simulink model "DYNctl_ver4_etud_obfusc2015"  (R2015a)
settings: Solver=ode45  StartTime=0.0  StopTime=tfin  FixedStep=0.001  RelTol=1e-09
values from neighbouring files (symbols this model uses):
  A = [line1;line2;line3;line4;line5]    [sm_7.m]
  B = [m0_3x3; m0_3x3; m0_2x3; m0_2x3; mCV_3x3]    [sm_7.m]
  C = [mTTdef m0_3x3 m0_3x4 m0_3x3 ... (first row only)    [sm_7.m]
  D = zeros(7,3)    [sm_7.m]
undefined symbols (not defined in the file or in its folder): ae0, ae1, ae2, ae3, as0, as1, as2, as3, be1, C_prime, D_prime, ia_e, ib_e, ic_e, phi_e, TABC_trans, TDEF_trans, theta_e, va_e, vb_e, vc_e, vx_s_e, vy_s_e, vz_e, w_phi_e, w_theta_e, x_s_e, y_s_e, z_e, za_e, zb_e, zc_e, zd_e, ze_e, zf_e
settings Model: CovSFcnEnable=off  Creator=delafontaine  LastModifiedBy=Sytten
settings SolverCC: AlgebraicLoopSolver=LineSearch
settings DataIOCC: SignalLoggingSaveFormat=ModelDataLogs
settings DebuggingCC: UnderspecifiedInitializationDetection=Classic  MergeDetectMultiDrivingBlocksExec=none  MultiTaskDSMMsg=warning  MultiTaskCondExecSysMsg=none

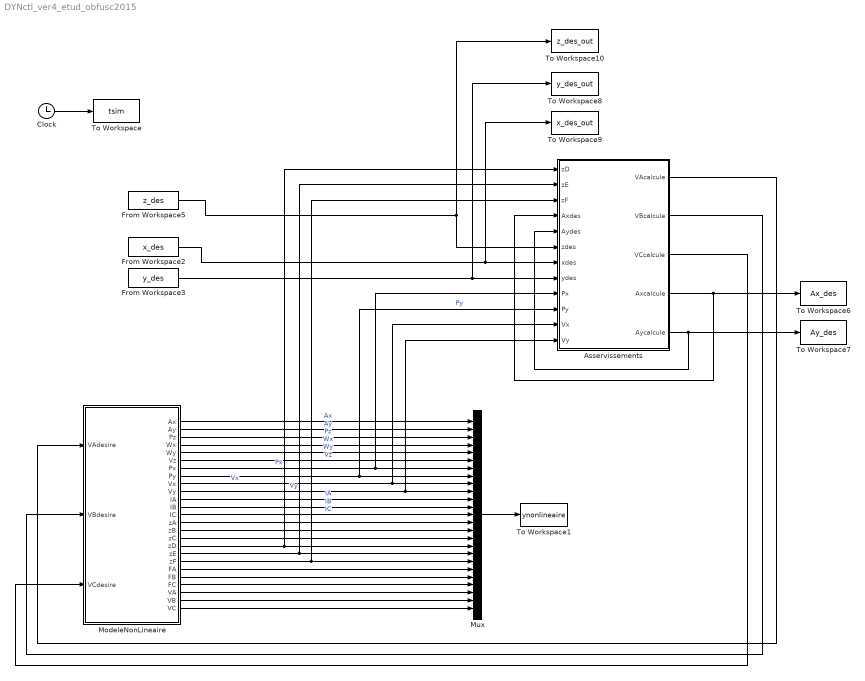
== system DYNctl_ver4_etud_obfusc2015 ==
  Asservissements : Subsystem
      mask help: Simulink:masks:GenSFuncDesc_MD
      mask Help: eval('feval(''rtwprivate'',''rtwhelpview'',''rtw_sfcn_block'')');
  Clock : Clock
  From Workspace2 : FromWorkspace  VariableName=x_des  SampleTime=0  Interpolate=off  OutputAfterFinalValue=Holding final value
  From Workspace3 : FromWorkspace  VariableName=y_des  SampleTime=0  Interpolate=off  OutputAfterFinalValue=Holding final value
  From Workspace5 : FromWorkspace  VariableName=z_des  SampleTime=0  Interpolate=off  OutputAfterFinalValue=Holding final value
  ModeleNonLineaire : Subsystem
      mask help: Simulink:masks:GenSFuncDesc_MD
      mask Help: eval('feval(''rtwprivate'',''rtwhelpview'',''rtw_sfcn_block'')');
  Mux : Mux  Inputs=25
  To Workspace : ToWorkspace  VariableName=tsim  SampleTime=-1
  To Workspace1 : ToWorkspace  VariableName=ynonlineaire  SampleTime=-1
  To Workspace10 : ToWorkspace  VariableName=z_des_out  SampleTime=-1
  To Workspace6 : ToWorkspace  VariableName=Ax_des  SampleTime=-1
  To Workspace7 : ToWorkspace  VariableName=Ay_des  SampleTime=-1
  To Workspace8 : ToWorkspace  VariableName=y_des_out  SampleTime=-1
  To Workspace9 : ToWorkspace  VariableName=x_des_out  SampleTime=-1
  wires:
  Mux/1 -> To Workspace1/1
  Clock/1 -> To Workspace/1
  From Workspace5/1 -> Asservissements/6(zdes), To Workspace10/1
  ModeleNonLineaire/1(Ax) -> Mux/1  "Ax"
  ModeleNonLineaire/2(Ay) -> Mux/2  "Ay"
  ModeleNonLineaire/3(Pz) -> Mux/3  "Pz"
  ModeleNonLineaire/4(Wx) -> Mux/4  "Wx"
  ModeleNonLineaire/5(Wy) -> Mux/5  "Wy"
  ModeleNonLineaire/6(Vz) -> Mux/6  "Vz"
  ModeleNonLineaire/7(Px) -> Asservissements/9(Px), Mux/7  "Px"
  ModeleNonLineaire/8(Py) -> Asservissements/10(Py), Mux/8  "Py"
  ModeleNonLineaire/9(Vx) -> Asservissements/11(Vx), Mux/9  "Vx"
  ModeleNonLineaire/10(Vy) -> Asservissements/12(Vy), Mux/10  "Vy"
  ModeleNonLineaire/11(IA) -> Mux/11  "IA"
  ModeleNonLineaire/12(IB) -> Mux/12  "IB"
  ModeleNonLineaire/13(IC) -> Mux/13  "IC"
  From Workspace3/1 -> Asservissements/8(ydes), To Workspace8/1
  From Workspace2/1 -> Asservissements/7(xdes), To Workspace9/1
  ModeleNonLineaire/20(FA) -> Mux/20
  ModeleNonLineaire/21(FB) -> Mux/21
  ModeleNonLineaire/22(FC) -> Mux/22
  ModeleNonLineaire/23(VA) -> Mux/23
  ModeleNonLineaire/24(VB) -> Mux/24
  ModeleNonLineaire/25(VC) -> Mux/25
  ModeleNonLineaire/17(zD) -> Asservissements/1(zD), Mux/17
  ModeleNonLineaire/18(zE) -> Asservissements/2(zE), Mux/18
  ModeleNonLineaire/19(zF) -> Asservissements/3(zF), Mux/19
  ModeleNonLineaire/14(zA) -> Mux/14
  ModeleNonLineaire/15(zB) -> Mux/15
  ModeleNonLineaire/16(zC) -> Mux/16
  Asservissements/4(Axcalcule) -> Asservissements/4(Axdes), To Workspace6/1
  Asservissements/5(Aycalcule) -> Asservissements/5(Aydes), To Workspace7/1
  Asservissements/1(VAcalcule) -> ModeleNonLineaire/1(VAdesire)
  Asservissements/2(VBcalcule) -> ModeleNonLineaire/2(VBdesire)
  Asservissements/3(VCcalcule) -> ModeleNonLineaire/3(VCdesire)

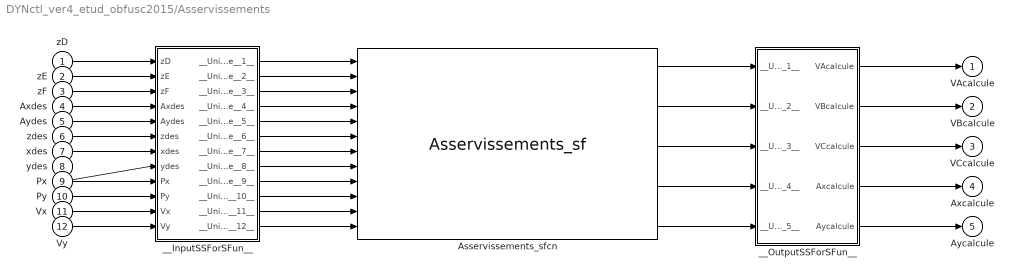
== system DYNctl_ver4_etud_obfusc2015/Asservissements ==
  zD : Inport
  zE : Inport  Port=2
  zF : Inport  Port=3
  Axdes : Inport  Port=4
  Aydes : Inport  Port=5
  zdes : Inport  Port=6
  xdes : Inport  Port=7
  ydes : Inport  Port=8
  Px : Inport  Port=9
  Py : Inport  Port=10
  Vx : Inport  Port=11
  Vy : Inport  Port=12
  Asservissements_sfcn : S-Function  FunctionName=Asservissements_sf  SFunctionModules=""  SFunctionDeploymentMode=off  EnableBusSupport=off  mask{rtw_sf_name=Asservissements_sf, showVar=off}
      mask prompts: rtw_sf_name "Simulink:masks:GenSFuncName_MP"; showVar "Simulink:masks:GenSFuncShowModuleList_MP"
      mask help: Simulink:masks:GenSFuncDesc_MD
      mask init:
      | displist = '';
      | if ~strcmp(get_param(gcb, 'FunctionName'), rtw_sf_name);
      |   set_param(gcb, 'FunctionName', rtw_sf_name);
      | end
      | % Check if we are generating code
      | rtw_mode = false;
      | if strcmpi(get_param(bdroot(gcb),'SimulationStatus'),'Initializing')
      | 	rtw_mode = strcmpi(get_param(bdroot(gcb),'BuildingRTWCode'),'on') && ...
      | 		~strcmpi(get_param(bdroot(gcb),'TargetStyle'),'SimulationTarget');
      | end
      | if showVar || rtw_mode
      | 	if exist('rtwsfunc') == 2 | exist('rtwsfunc') == 6
      | 		tmplist = rtwsfunc(rtw_sf_name,gcb);
      | 		tmplist = DAStudio.message('Simulink:masks:GenSFuncListOfModules_IC', tmplist);
      | 	elseif showVar
      | 		tmplist1 = DAStudio.message('Simulink:masks:GenSFuncListOfModules_IC', '');
      |         tmplist2 = DAStudio.message('Simulink:masks:GenSFuncNotLicensed_IC');
      |         tmplist = [tmplist1 tmplist2];
      |  	end
      | end
      | if showVar
      |   displist = tmplist;
      | end
      settings: CopyFcn=|
      | if ~strcmp(get_param(gcb,'Linkstatus'),'none') && ...
      | ~strcmp(get_param(gcb,'Linkstatus'),'implicit')
      |   set_param(gcb,'LinkStatus','none');
      | end
      mask Help: eval('feval(''rtwprivate'',''rtwhelpview'',''rtw_sfcn_block'')');
      mask Display:
      | port_label('input',1,'zD');
      | port_label('input',2,'zE');
      | port_label('input',3,'zF');
      | port_label('input',4,'Axdes');
      | port_label('input',5,'Aydes');
      | port_label('input',6,'zdes');
      | port_label('input',7,'xdes');
      | port_label('input',8,'ydes');
      | port_label('input',9,'Px');
      | port_label('input',10,'Py');
      | port_label('input',11,'Vx');
      | port_label('input',12,'Vy');
      | port_label('output',1,'VAcalcule');
      | port_label('output',2,'VBcalcule');
      | port_label('output',3,'VCcalcule');
      | port_label('output',4,'Axcalcule');
      | port_label('output',5,'Aycalcule');
  __InputSSForSFun__ : Subsystem
      settings: PermitHierarchicalResolution=ParametersOnly
  __OutputSSForSFun__ : Subsystem
      settings: PermitHierarchicalResolution=ParametersOnly
  VAcalcule : Outport
  VBcalcule : Outport  Port=2
  VCcalcule : Outport  Port=3
  Axcalcule : Outport  Port=4
  Aycalcule : Outport  Port=5
  wires:
  zD/1 -> __InputSSForSFun__/1(zD)
  zE/1 -> __InputSSForSFun__/2(zE)
  zF/1 -> __InputSSForSFun__/3(zF)
  Axdes/1 -> __InputSSForSFun__/4(Axdes)
  Aydes/1 -> __InputSSForSFun__/5(Aydes)
  zdes/1 -> __InputSSForSFun__/6(zdes)
  xdes/1 -> __InputSSForSFun__/7(xdes)
  ydes/1 -> __InputSSForSFun__/8(ydes)
  Px/1 -> __InputSSForSFun__/9(Px)
  Py/1 -> __InputSSForSFun__/10(Py)
  Vx/1 -> __InputSSForSFun__/11(Vx)
  Vy/1 -> __InputSSForSFun__/12(Vy)
  __InputSSForSFun__/1(__UniqueOutportName__1__) -> Asservissements_sfcn/1
  __InputSSForSFun__/2(__UniqueOutportName__2__) -> Asservissements_sfcn/2
  __InputSSForSFun__/3(__UniqueOutportName__3__) -> Asservissements_sfcn/3
  __InputSSForSFun__/4(__UniqueOutportName__4__) -> Asservissements_sfcn/4
  __InputSSForSFun__/5(__UniqueOutportName__5__) -> Asservissements_sfcn/5
  __InputSSForSFun__/6(__UniqueOutportName__6__) -> Asservissements_sfcn/6
  __InputSSForSFun__/7(__UniqueOutportName__7__) -> Asservissements_sfcn/7
  __InputSSForSFun__/8(__UniqueOutportName__8__) -> Asservissements_sfcn/8
  __InputSSForSFun__/9(__UniqueOutportName__9__) -> Asservissements_sfcn/9
  __InputSSForSFun__/10(__UniqueOutportName__10__) -> Asservissements_sfcn/10
  __InputSSForSFun__/11(__UniqueOutportName__11__) -> Asservissements_sfcn/11
  __InputSSForSFun__/12(__UniqueOutportName__12__) -> Asservissements_sfcn/12
  Asservissements_sfcn/1 -> __OutputSSForSFun__/1(__UniqueInportName__1__)
  Asservissements_sfcn/2 -> __OutputSSForSFun__/2(__UniqueInportName__2__)
  Asservissements_sfcn/3 -> __OutputSSForSFun__/3(__UniqueInportName__3__)
  Asservissements_sfcn/4 -> __OutputSSForSFun__/4(__UniqueInportName__4__)
  Asservissements_sfcn/5 -> __OutputSSForSFun__/5(__UniqueInportName__5__)
  __OutputSSForSFun__/1(VAcalcule) -> VAcalcule/1
  __OutputSSForSFun__/2(VBcalcule) -> VBcalcule/1
  __OutputSSForSFun__/3(VCcalcule) -> VCcalcule/1
  __OutputSSForSFun__/4(Axcalcule) -> Axcalcule/1
  __OutputSSForSFun__/5(Aycalcule) -> Aycalcule/1

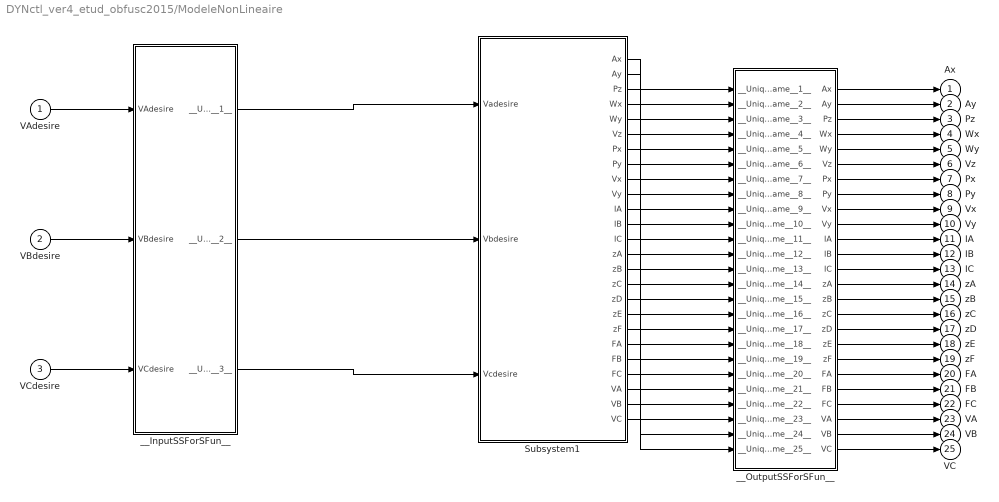
== system DYNctl_ver4_etud_obfusc2015/ModeleNonLineaire ==
  VAdesire : Inport
  VBdesire : Inport  Port=2
  VCdesire : Inport  Port=3
  Subsystem1 : Subsystem
  __InputSSForSFun__ : Subsystem
      settings: PermitHierarchicalResolution=ParametersOnly
  __OutputSSForSFun__ : Subsystem
      settings: PermitHierarchicalResolution=ParametersOnly
  Ax : Outport
  Ay : Outport  Port=2
  Pz : Outport  Port=3
  Wx : Outport  Port=4
  Wy : Outport  Port=5
  Vz : Outport  Port=6
  Px : Outport  Port=7
  Py : Outport  Port=8
  Vx : Outport  Port=9
  Vy : Outport  Port=10
  IA : Outport  Port=11
  IB : Outport  Port=12
  IC : Outport  Port=13
  zA : Outport  Port=14
  zB : Outport  Port=15
  zC : Outport  Port=16
  zD : Outport  Port=17
  zE : Outport  Port=18
  zF : Outport  Port=19
  FA : Outport  Port=20
  FB : Outport  Port=21
  FC : Outport  Port=22
  VA : Outport  Port=23
  VB : Outport  Port=24
  VC : Outport  Port=25
  wires:
  VAdesire/1 -> __InputSSForSFun__/1(VAdesire)
  VBdesire/1 -> __InputSSForSFun__/2(VBdesire)
  VCdesire/1 -> __InputSSForSFun__/3(VCdesire)
  Subsystem1/1(Ax) -> __OutputSSForSFun__/1(__UniqueInportName__1__)
  Subsystem1/2(Ay) -> __OutputSSForSFun__/2(__UniqueInportName__2__)
  Subsystem1/3(Pz) -> __OutputSSForSFun__/3(__UniqueInportName__3__)
  Subsystem1/4(Wx) -> __OutputSSForSFun__/4(__UniqueInportName__4__)
  Subsystem1/5(Wy) -> __OutputSSForSFun__/5(__UniqueInportName__5__)
  Subsystem1/6(Vz) -> __OutputSSForSFun__/6(__UniqueInportName__6__)
  Subsystem1/7(Px) -> __OutputSSForSFun__/7(__UniqueInportName__7__)
  Subsystem1/8(Py) -> __OutputSSForSFun__/8(__UniqueInportName__8__)
  Subsystem1/9(Vx) -> __OutputSSForSFun__/9(__UniqueInportName__9__)
  Subsystem1/10(Vy) -> __OutputSSForSFun__/10(__UniqueInportName__10__)
  Subsystem1/11(IA) -> __OutputSSForSFun__/11(__UniqueInportName__11__)
  Subsystem1/12(IB) -> __OutputSSForSFun__/12(__UniqueInportName__12__)
  Subsystem1/13(IC) -> __OutputSSForSFun__/13(__UniqueInportName__13__)
  Subsystem1/14(zA) -> __OutputSSForSFun__/14(__UniqueInportName__14__)
  Subsystem1/15(zB) -> __OutputSSForSFun__/15(__UniqueInportName__15__)
  Subsystem1/16(zC) -> __OutputSSForSFun__/16(__UniqueInportName__16__)
  Subsystem1/17(zD) -> __OutputSSForSFun__/17(__UniqueInportName__17__)
  Subsystem1/18(zE) -> __OutputSSForSFun__/18(__UniqueInportName__18__)
  Subsystem1/19(zF) -> __OutputSSForSFun__/19(__UniqueInportName__19__)
  Subsystem1/20(FA) -> __OutputSSForSFun__/20(__UniqueInportName__20__)
  Subsystem1/21(FB) -> __OutputSSForSFun__/21(__UniqueInportName__21__)
  Subsystem1/22(FC) -> __OutputSSForSFun__/22(__UniqueInportName__22__)
  Subsystem1/23(VA) -> __OutputSSForSFun__/23(__UniqueInportName__23__)
  Subsystem1/24(VB) -> __OutputSSForSFun__/24(__UniqueInportName__24__)
  Subsystem1/25(VC) -> __OutputSSForSFun__/25(__UniqueInportName__25__)
  __OutputSSForSFun__/1(Ax) -> Ax/1
  __OutputSSForSFun__/2(Ay) -> Ay/1
  __OutputSSForSFun__/3(Pz) -> Pz/1
  __OutputSSForSFun__/4(Wx) -> Wx/1
  __OutputSSForSFun__/5(Wy) -> Wy/1
  __OutputSSForSFun__/6(Vz) -> Vz/1
  __OutputSSForSFun__/7(Px) -> Px/1
  __OutputSSForSFun__/8(Py) -> Py/1
  __OutputSSForSFun__/9(Vx) -> Vx/1
  __OutputSSForSFun__/10(Vy) -> Vy/1
  __OutputSSForSFun__/11(IA) -> IA/1
  __OutputSSForSFun__/12(IB) -> IB/1
  __OutputSSForSFun__/13(IC) -> IC/1
  __OutputSSForSFun__/14(zA) -> zA/1
  __OutputSSForSFun__/15(zB) -> zB/1
  __OutputSSForSFun__/16(zC) -> zC/1
  __OutputSSForSFun__/17(zD) -> zD/1
  __OutputSSForSFun__/18(zE) -> zE/1
  __OutputSSForSFun__/19(zF) -> zF/1
  __OutputSSForSFun__/20(FA) -> FA/1
  __OutputSSForSFun__/21(FB) -> FB/1
  __OutputSSForSFun__/22(FC) -> FC/1
  __OutputSSForSFun__/23(VA) -> VA/1
  __OutputSSForSFun__/24(VB) -> VB/1
  __OutputSSForSFun__/25(VC) -> VC/1
  __InputSSForSFun__/1(__UniqueOutportName__1__) -> Subsystem1/1(Vadesire)
  __InputSSForSFun__/2(__UniqueOutportName__2__) -> Subsystem1/2(Vbdesire)
  __InputSSForSFun__/3(__UniqueOutportName__3__) -> Subsystem1/3(Vcdesire)

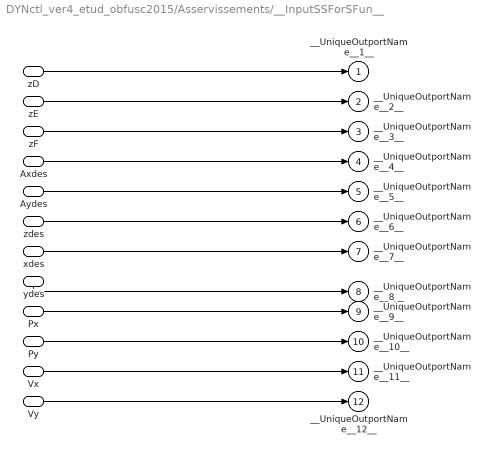
== system DYNctl_ver4_etud_obfusc2015/Asservissements/__InputSSForSFun__ ==
  zD : Inport
  zE : Inport  Port=2
  zF : Inport  Port=3
  Axdes : Inport  Port=4
  Aydes : Inport  Port=5
  zdes : Inport  Port=6
  xdes : Inport  Port=7
  ydes : Inport  Port=8
  Px : Inport  Port=9
  Py : Inport  Port=10
  Vx : Inport  Port=11
  Vy : Inport  Port=12
  __UniqueOutportName__1__ : Outport
  __UniqueOutportName__2__ : Outport  Port=2
  __UniqueOutportName__3__ : Outport  Port=3
  __UniqueOutportName__4__ : Outport  Port=4
  __UniqueOutportName__5__ : Outport  Port=5
  __UniqueOutportName__6__ : Outport  Port=6
  __UniqueOutportName__7__ : Outport  Port=7
  __UniqueOutportName__8__ : Outport  Port=8
  __UniqueOutportName__9__ : Outport  Port=9
  __UniqueOutportName__10__ : Outport  Port=10
  __UniqueOutportName__11__ : Outport  Port=11
  __UniqueOutportName__12__ : Outport  Port=12
  wires:
  zD/1 -> __UniqueOutportName__1__/1
  zE/1 -> __UniqueOutportName__2__/1
  zF/1 -> __UniqueOutportName__3__/1
  Axdes/1 -> __UniqueOutportName__4__/1
  Aydes/1 -> __UniqueOutportName__5__/1
  zdes/1 -> __UniqueOutportName__6__/1
  xdes/1 -> __UniqueOutportName__7__/1
  ydes/1 -> __UniqueOutportName__8__/1
  Px/1 -> __UniqueOutportName__9__/1
  Py/1 -> __UniqueOutportName__10__/1
  Vx/1 -> __UniqueOutportName__11__/1
  Vy/1 -> __UniqueOutportName__12__/1

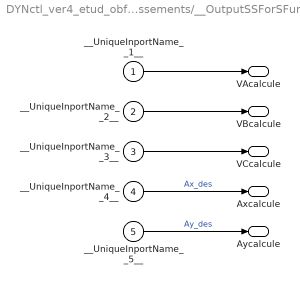
== system DYNctl_ver4_etud_obfusc2015/Asservissements/__OutputSSForSFun__ ==
  __UniqueInportName__1__ : Inport
  __UniqueInportName__2__ : Inport  Port=2
  __UniqueInportName__3__ : Inport  Port=3
  __UniqueInportName__4__ : Inport  Port=4
  __UniqueInportName__5__ : Inport  Port=5
  VAcalcule : Outport
  VBcalcule : Outport  Port=2
  VCcalcule : Outport  Port=3
  Axcalcule : Outport  Port=4
  Aycalcule : Outport  Port=5
  wires:
  __UniqueInportName__1__/1 -> VAcalcule/1
  __UniqueInportName__2__/1 -> VBcalcule/1
  __UniqueInportName__3__/1 -> VCcalcule/1
  __UniqueInportName__4__/1 -> Axcalcule/1  "Ax_des"
  __UniqueInportName__5__/1 -> Aycalcule/1  "Ay_des"

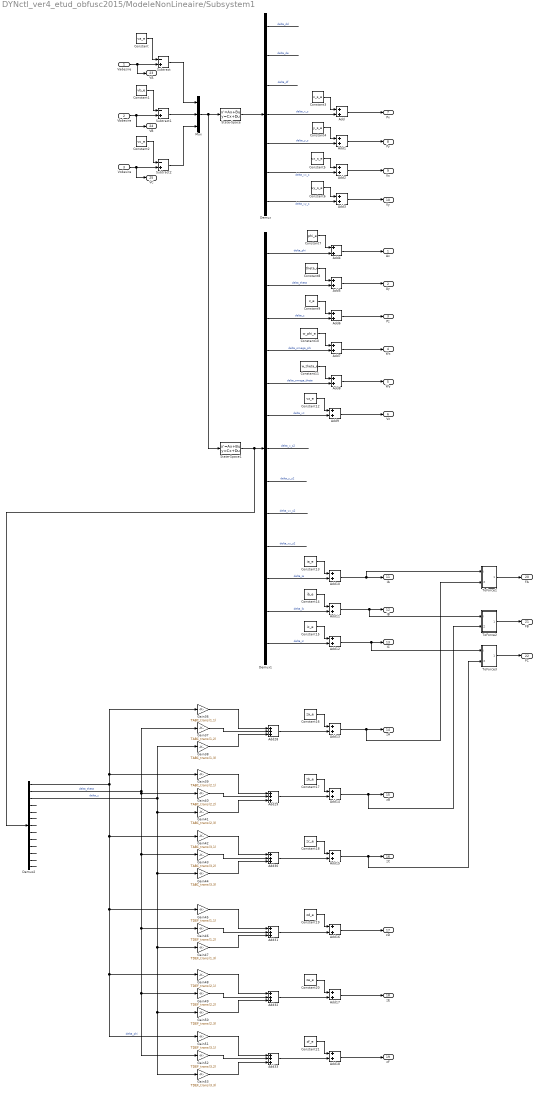
== system DYNctl_ver4_etud_obfusc2015/ModeleNonLineaire/Subsystem1 ==
  Vadesire : Inport
  Vbdesire : Inport  Port=2
  Vcdesire : Inport  Port=3
  Add{,1..18} (19 alike) : Sum
  Add{28..33} (6 alike) : Sum  Inputs=+++
  Constant : Constant  Value=va_e
  Constant1 : Constant  Value=vb_e
  Constant10 : Constant  Value=w_phi_e
  Constant11 : Constant  Value=w_theta_e
  Constant12 : Constant  Value=vz_e
  Constant13 : Constant  Value=ia_e
  Constant14 : Constant  Value=ib_e
  Constant15 : Constant  Value=ic_e
  Constant16 : Constant  Value=za_e
  Constant17 : Constant  Value=zb_e
  Constant18 : Constant  Value=zc_e
  Constant19 : Constant  Value=zd_e
  Constant2 : Constant  Value=vc_e
  Constant20 : Constant  Value=ze_e
  Constant21 : Constant  Value=zf_e
  Constant3 : Constant  Value=x_s_e
  Constant4 : Constant  Value=y_s_e
  Constant5 : Constant  Value=vx_s_e
  Constant6 : Constant  Value=vy_s_e
  Constant7 : Constant  Value=phi_e
  Constant8 : Constant  Value=theta_e
  Constant9 : Constant  Value=z_e
  Demux : Demux  Outputs=7
  Demux1 : Demux  Outputs=13
  Demux2 : Demux  Outputs=13
  Gain36 : Gain  Gain=TABC_trans(1,1)
  Gain37 : Gain  Gain=TABC_trans(1,2)
  Gain38 : Gain  Gain=TABC_trans(1,3)
  Gain39 : Gain  Gain=TABC_trans(2,1)
  Gain40 : Gain  Gain=TABC_trans(2,2)
  Gain41 : Gain  Gain=TABC_trans(2,3)
  Gain42 : Gain  Gain=TABC_trans(3,1)
  Gain43 : Gain  Gain=TABC_trans(3,2)
  Gain44 : Gain  Gain=TABC_trans(3,3)
  Gain45 : Gain  Gain=TDEF_trans(1,1)
  Gain46 : Gain  Gain=TDEF_trans(1,2)
  Gain47 : Gain  Gain=TDEF_trans(1,3)
  Gain48 : Gain  Gain=TDEF_trans(2,1)
  Gain49 : Gain  Gain=TDEF_trans(2,2)
  Gain50 : Gain  Gain=TDEF_trans(2,3)
  Gain51 : Gain  Gain=TDEF_trans(3,1)
  Gain52 : Gain  Gain=TDEF_trans(3,2)
  Gain53 : Gain  Gain=TDEF_trans(3,3)
  Mux : Mux  Inputs=3
  State-Space : StateSpace  A=A  B=B  C=C  D=D  X0=0
  State-Space1 : StateSpace  A=A  B=B  C=C_prime  D=D_prime  X0=0
  Subtract : Sum  Inputs=-+
  Subtract1 : Sum  Inputs=-+
  Subtract2 : Sum  Inputs=-+
  ToForce1 : Subsystem
  ToForce2 : Subsystem
  ToForce3 : Subsystem
  Ax : Outport
  Ay : Outport  Port=2
  Pz : Outport  Port=3
  Wx : Outport  Port=4
  Wy : Outport  Port=5
  Vz : Outport  Port=6
  Px : Outport  Port=7
  Py : Outport  Port=8
  Vx : Outport  Port=9
  Vy : Outport  Port=10
  IA : Outport  Port=11
  IB : Outport  Port=12
  IC : Outport  Port=13
  zA : Outport  Port=14
  zB : Outport  Port=15
  zC : Outport  Port=16
  zD : Outport  Port=17
  zE : Outport  Port=18
  zF : Outport  Port=19
  FA : Outport  Port=20
  FB : Outport  Port=21
  FC : Outport  Port=22
  VA : Outport  Port=23
  VB : Outport  Port=24
  VC : Outport  Port=25
  wires:
  Demux2/6 -> ?
  Demux2/11 -> ?
  Add11/1 -> ToForce2/1(I), IB/1
  Demux2/7 -> ?
  Demux2/13 -> ?
  Gain44/1 -> Add30/3
  Constant13/1 -> Add10/1
  Constant15/1 -> Add12/1
  Gain50/1 -> Add32/3
  Demux1/13 -> Add12/2  "delta_ic"
  Demux1/7 -> ?  "delta_x_s2"
  Gain52/1 -> Add33/2
  Gain36/1 -> Add28/1
  Constant14/1 -> Add11/1
  Demux2/1 -> Gain48/1, Gain51/1, Gain45/1, Gain42/1, Gain39/1, Gain36/1  "delta_phi"
  Gain38/1 -> Add28/3
  Demux2/2 -> Gain37/1, Gain40/1, Gain52/1, Gain49/1, Gain46/1, Gain43/1  "delta_theta"
  Constant18/1 -> Add15/1
  Add28/1 -> Add13/2
  Add29/1 -> Add14/2
  Demux1/1 -> Add4/2  "delta_phi"
  Gain39/1 -> Add29/1
  Constant16/1 -> Add13/1
  Add30/1 -> Add15/2
  Constant11/1 -> Add8/1
  Demux1/4 -> Add7/2  "delta_omega_phi"
  Add2/1 -> Vx/1
  State-Space1/1 -> Demux2/1, Demux1/1
  Constant1/1 -> Subtract1/1
  Add1/1 -> Py/1
  Demux/2 -> ?  "delta_de"
  Vadesire/1 -> VA/1, Subtract/2
  Add3/1 -> Vy/1
  Constant17/1 -> Add14/1
  Constant4/1 -> Add1/1
  Constant3/1 -> Add/1
  Demux/4 -> Add/2  "delta_x_s"
  Demux/3 -> ?  "delta_df"
  Add9/1 -> Vz/1
  Constant12/1 -> Add9/1
  Constant5/1 -> Add2/1
  Demux1/6 -> Add9/2  "delta_vz"
  Demux1/10 -> ?  "delta_vy_s2"
  Vcdesire/1 -> VC/1, Subtract2/2
  Subtract1/1 -> Mux/2
  Add8/1 -> Wy/1
  Constant2/1 -> Subtract2/1
  Constant6/1 -> Add3/1
  Subtract2/1 -> Mux/3
  Add16/1 -> zD/1
  Add17/1 -> zE/1
  State-Space/1 -> Demux/1
  Gain53/1 -> Add33/3
  Demux1/9 -> ?  "delta_vx_s2"
  Demux2/10 -> ?
  Add33/1 -> Add18/2
  Demux/1 -> ?  "delta_dd"
  Subtract/1 -> Mux/1
  Demux/5 -> Add1/2  "delta_y_s"
  Add13/1 -> ToForce1/2(Z), zA/1
  Gain48/1 -> Add32/1
  Gain51/1 -> Add33/1
  Add15/1 -> ToForce3/2(Z), zC/1
  Add7/1 -> Wx/1
  Gain47/1 -> Add31/3
  Add14/1 -> ToForce2/2(Z), zB/1
  Constant10/1 -> Add7/1
  Add18/1 -> zF/1
  Gain43/1 -> Add30/2
  Demux2/3 -> Gain53/1, Gain50/1, Gain47/1, Gain44/1, Gain41/1, Gain38/1  "delta_z"
  Constant/1 -> Subtract/1
  Constant19/1 -> Add16/1
  Add32/1 -> Add17/2
  Add31/1 -> Add16/2
  Gain42/1 -> Add30/1
  Gain41/1 -> Add29/3
  Demux1/2 -> Add5/2  "delta_theta"
  Gain49/1 -> Add32/2
  Mux/1 -> State-Space1/1, State-Space/1
  Demux1/8 -> ?  "delta_y_s2"
  Demux/7 -> Add3/2  "delta_vy_s"
  Constant20/1 -> Add17/1
  Gain40/1 -> Add29/2
  Demux1/5 -> Add8/2  "delta_omega_theta"
  Demux2/4 -> ?
  Demux2/9 -> ?
  Demux2/8 -> ?
  Demux2/5 -> ?
  Demux1/12 -> Add11/2  "delta_ib"
  Vbdesire/1 -> VB/1, Subtract1/2
  Add/1 -> Px/1
  Demux/6 -> Add2/2  "delta_vx_s"
  Gain37/1 -> Add28/2
  Constant7/1 -> Add4/1
  Constant9/1 -> Add6/1
  Add5/1 -> Ay/1
  Add12/1 -> ToForce3/1(I), IC/1
  Demux1/3 -> Add6/2  "delta_z"
  Add6/1 -> Pz/1
  Constant8/1 -> Add5/1
  Gain46/1 -> Add31/2
  Demux1/11 -> Add10/2  "delta_ia"
  Gain45/1 -> Add31/1
  Add4/1 -> Ax/1
  Add10/1 -> ToForce1/1(I), IA/1
  Constant21/1 -> Add18/1
  Demux2/12 -> ?
  ToForce1/1(Force) -> FA/1
  ToForce2/1(Force) -> FB/1
  ToForce3/1(Force) -> FC/1

== system DYNctl_ver4_etud_obfusc2015/ModeleNonLineaire/__InputSSForSFun__ ==
  VAdesire : Inport
  VBdesire : Inport  Port=2
  VCdesire : Inport  Port=3
  __UniqueOutportName__1__ : Outport
  __UniqueOutportName__2__ : Outport  Port=2
  __UniqueOutportName__3__ : Outport  Port=3
  wires:
  VAdesire/1 -> __UniqueOutportName__1__/1
  VBdesire/1 -> __UniqueOutportName__2__/1
  VCdesire/1 -> __UniqueOutportName__3__/1

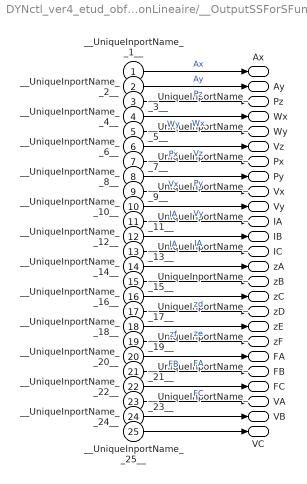
== system DYNctl_ver4_etud_obfusc2015/ModeleNonLineaire/__OutputSSForSFun__ ==
  __UniqueInportName__1__ : Inport
  __UniqueInportName__2__ : Inport  Port=2
  __UniqueInportName__3__ : Inport  Port=3
  __UniqueInportName__4__ : Inport  Port=4
  __UniqueInportName__5__ : Inport  Port=5
  __UniqueInportName__6__ : Inport  Port=6
  __UniqueInportName__7__ : Inport  Port=7
  __UniqueInportName__8__ : Inport  Port=8
  __UniqueInportName__9__ : Inport  Port=9
  __UniqueInportName__10__ : Inport  Port=10
  __UniqueInportName__11__ : Inport  Port=11
  __UniqueInportName__12__ : Inport  Port=12
  __UniqueInportName__13__ : Inport  Port=13
  __UniqueInportName__14__ : Inport  Port=14
  __UniqueInportName__15__ : Inport  Port=15
  __UniqueInportName__16__ : Inport  Port=16
  __UniqueInportName__17__ : Inport  Port=17
  __UniqueInportName__18__ : Inport  Port=18
  __UniqueInportName__19__ : Inport  Port=19
  __UniqueInportName__20__ : Inport  Port=20
  __UniqueInportName__21__ : Inport  Port=21
  __UniqueInportName__22__ : Inport  Port=22
  __UniqueInportName__23__ : Inport  Port=23
  __UniqueInportName__24__ : Inport  Port=24
  __UniqueInportName__25__ : Inport  Port=25
  Ax : Outport
  Ay : Outport  Port=2
  Pz : Outport  Port=3
  Wx : Outport  Port=4
  Wy : Outport  Port=5
  Vz : Outport  Port=6
  Px : Outport  Port=7
  Py : Outport  Port=8
  Vx : Outport  Port=9
  Vy : Outport  Port=10
  IA : Outport  Port=11
  IB : Outport  Port=12
  IC : Outport  Port=13
  zA : Outport  Port=14
  zB : Outport  Port=15
  zC : Outport  Port=16
  zD : Outport  Port=17
  zE : Outport  Port=18
  zF : Outport  Port=19
  FA : Outport  Port=20
  FB : Outport  Port=21
  FC : Outport  Port=22
  VA : Outport  Port=23
  VB : Outport  Port=24
  VC : Outport  Port=25
  wires:
  __UniqueInportName__1__/1 -> Ax/1  "Ax"
  __UniqueInportName__2__/1 -> Ay/1  "Ay"
  __UniqueInportName__3__/1 -> Pz/1  "Pz"
  __UniqueInportName__4__/1 -> Wx/1  "Wx"
  __UniqueInportName__5__/1 -> Wy/1  "Wy"
  __UniqueInportName__6__/1 -> Vz/1  "Vz"
  __UniqueInportName__7__/1 -> Px/1  "Px"
  __UniqueInportName__8__/1 -> Py/1  "Py"
  __UniqueInportName__9__/1 -> Vx/1  "Vx"
  __UniqueInportName__10__/1 -> Vy/1  "Vy"
  __UniqueInportName__11__/1 -> IA/1  "IA"
  __UniqueInportName__12__/1 -> IB/1  "IA"
  __UniqueInportName__13__/1 -> IC/1  "IA"
  __UniqueInportName__14__/1 -> zA/1
  __UniqueInportName__15__/1 -> zB/1
  __UniqueInportName__16__/1 -> zC/1
  __UniqueInportName__17__/1 -> zD/1  "zd"
  __UniqueInportName__18__/1 -> zE/1  "ze"
  __UniqueInportName__19__/1 -> zF/1  "zf"
  __UniqueInportName__20__/1 -> FA/1  "FA"
  __UniqueInportName__21__/1 -> FB/1  "FB"
  __UniqueInportName__22__/1 -> FC/1  "FC"
  __UniqueInportName__23__/1 -> VA/1
  __UniqueInportName__24__/1 -> VB/1
  __UniqueInportName__25__/1 -> VC/1

== system DYNctl_ver4_etud_obfusc2015/ModeleNonLineaire/Subsystem1/ToForce1 ==
  I : Inport
  Z : Inport  Port=2
  Add35 : Sum
  Divide2 : Product  Inputs=*/
  Subsystem : Subsystem
  Subsystem1 : Subsystem
  Force : Outport
  wires:
  Subsystem1/1(Out1) -> Divide2/1
  Z/1 -> Subsystem/1(In1)
  Subsystem/2(Out2) -> Divide2/2
  Divide2/1 -> Add35/1
  Add35/1 -> Force/1
  I/1 -> Subsystem1/1(In1)
  Subsystem/1(Out1) -> Add35/2

== system DYNctl_ver4_etud_obfusc2015/ModeleNonLineaire/Subsystem1/ToForce2 ==
  I : Inport
  Z : Inport  Port=2
  Add35 : Sum
  Divide2 : Product  Inputs=*/
  Subsystem : Subsystem
  Subsystem1 : Subsystem
  Force : Outport
  wires:
  Subsystem1/1(Out1) -> Divide2/1
  Z/1 -> Subsystem/1(In1)
  Subsystem/2(Out2) -> Divide2/2
  Divide2/1 -> Add35/1
  Add35/1 -> Force/1
  I/1 -> Subsystem1/1(In1)
  Subsystem/1(Out1) -> Add35/2

== system DYNctl_ver4_etud_obfusc2015/ModeleNonLineaire/Subsystem1/ToForce3 ==
  I : Inport
  Z : Inport  Port=2
  Add35 : Sum
  Divide2 : Product  Inputs=*/
  Subsystem : Subsystem
  Subsystem1 : Subsystem
  Force : Outport
  wires:
  Subsystem1/1(Out1) -> Divide2/1
  Z/1 -> Subsystem/1(In1)
  Subsystem/2(Out2) -> Divide2/2
  Divide2/1 -> Add35/1
  Add35/1 -> Force/1
  I/1 -> Subsystem1/1(In1)
  Subsystem/1(Out1) -> Add35/2

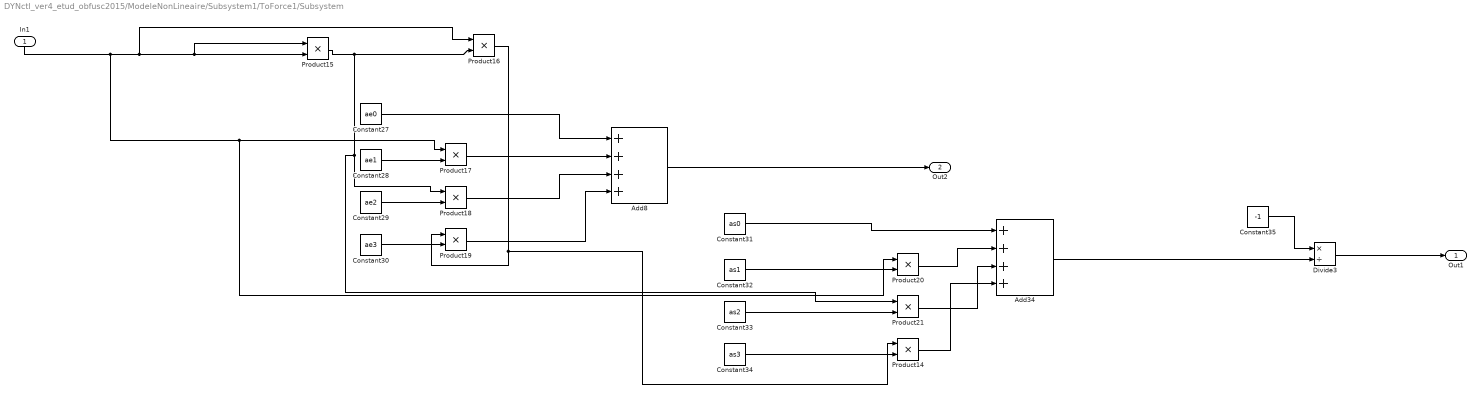
== system DYNctl_ver4_etud_obfusc2015/ModeleNonLineaire/Subsystem1/ToForce1/Subsystem ==
  In1 : Inport
  Add34 : Sum  Inputs=++++
  Add8 : Sum  Inputs=++++
  Constant27 : Constant  Value=ae0
  Constant28 : Constant  Value=ae1
  Constant29 : Constant  Value=ae2
  Constant30 : Constant  Value=ae3
  Constant31 : Constant  Value=as0
  Constant32 : Constant  Value=as1
  Constant33 : Constant  Value=as2
  Constant34 : Constant  Value=as3
  Constant35 : Constant  Value=-1
  Divide3 : Product  Inputs=*/
  Product{14..21} (8 alike) : Product
  Out1 : Outport
  Out2 : Outport  Port=2
  wires:
  In1/1 -> Product20/1, Product17/1, Product16/1, Product15/1, Product15/2
  Constant28/1 -> Product17/2
  Constant30/1 -> Product19/2
  Constant29/1 -> Product18/2
  Product15/1 -> Product21/1, Product18/1, Product16/2
  Product16/1 -> Product19/1, Product14/1
  Constant27/1 -> Add8/1
  Product17/1 -> Add8/2
  Product18/1 -> Add8/3
  Product19/1 -> Add8/4
  Add8/1 -> Out2/1
  Constant34/1 -> Product14/2
  Constant32/1 -> Product20/2
  Constant33/1 -> Product21/2
  Product20/1 -> Add34/2
  Product21/1 -> Add34/3
  Product14/1 -> Add34/4
  Constant31/1 -> Add34/1
  Add34/1 -> Divide3/2
  Constant35/1 -> Divide3/1
  Divide3/1 -> Out1/1

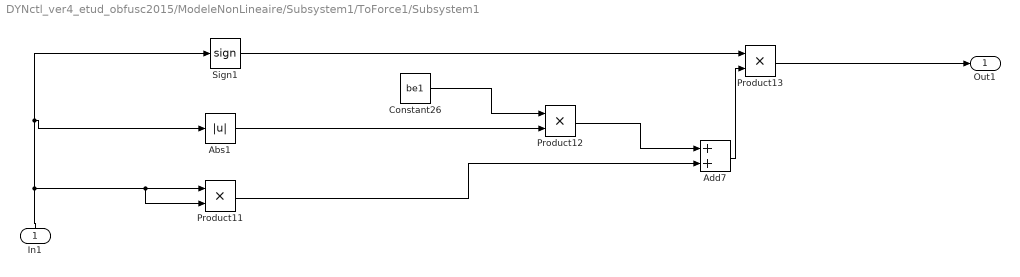
== system DYNctl_ver4_etud_obfusc2015/ModeleNonLineaire/Subsystem1/ToForce1/Subsystem1 ==
  In1 : Inport
  Abs1 : Abs
  Add7 : Sum
  Constant26 : Constant  Value=be1
  Product11 : Product
  Product12 : Product
  Product13 : Product
  Sign1 : Signum
  Out1 : Outport
  wires:
  In1/1 -> Abs1/1, Sign1/1, Product11/2, Product11/1
  Constant26/1 -> Product12/1
  Abs1/1 -> Product12/2
  Product12/1 -> Add7/1
  Product11/1 -> Add7/2
  Add7/1 -> Product13/2
  Product13/1 -> Out1/1
  Sign1/1 -> Product13/1

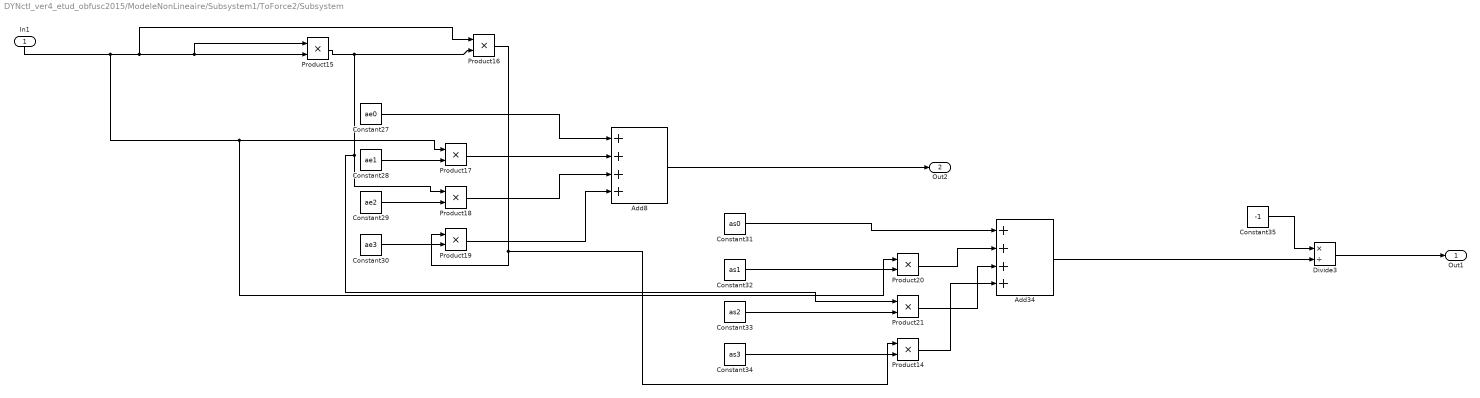
== system DYNctl_ver4_etud_obfusc2015/ModeleNonLineaire/Subsystem1/ToForce2/Subsystem ==
  In1 : Inport
  Add34 : Sum  Inputs=++++
  Add8 : Sum  Inputs=++++
  Constant27 : Constant  Value=ae0
  Constant28 : Constant  Value=ae1
  Constant29 : Constant  Value=ae2
  Constant30 : Constant  Value=ae3
  Constant31 : Constant  Value=as0
  Constant32 : Constant  Value=as1
  Constant33 : Constant  Value=as2
  Constant34 : Constant  Value=as3
  Constant35 : Constant  Value=-1
  Divide3 : Product  Inputs=*/
  Product{14..21} (8 alike) : Product
  Out1 : Outport
  Out2 : Outport  Port=2
  wires:
  In1/1 -> Product20/1, Product17/1, Product16/1, Product15/1, Product15/2
  Constant28/1 -> Product17/2
  Constant30/1 -> Product19/2
  Constant29/1 -> Product18/2
  Product15/1 -> Product21/1, Product18/1, Product16/2
  Product16/1 -> Product19/1, Product14/1
  Constant27/1 -> Add8/1
  Product17/1 -> Add8/2
  Product18/1 -> Add8/3
  Product19/1 -> Add8/4
  Add8/1 -> Out2/1
  Constant34/1 -> Product14/2
  Constant32/1 -> Product20/2
  Constant33/1 -> Product21/2
  Product20/1 -> Add34/2
  Product21/1 -> Add34/3
  Product14/1 -> Add34/4
  Constant31/1 -> Add34/1
  Add34/1 -> Divide3/2
  Constant35/1 -> Divide3/1
  Divide3/1 -> Out1/1

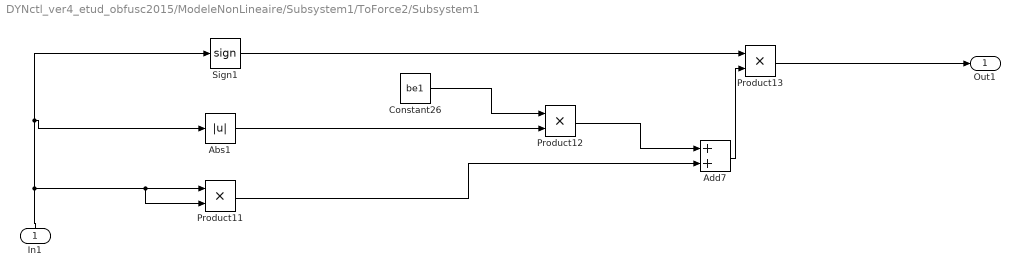
== system DYNctl_ver4_etud_obfusc2015/ModeleNonLineaire/Subsystem1/ToForce2/Subsystem1 ==
  In1 : Inport
  Abs1 : Abs
  Add7 : Sum
  Constant26 : Constant  Value=be1
  Product11 : Product
  Product12 : Product
  Product13 : Product
  Sign1 : Signum
  Out1 : Outport
  wires:
  In1/1 -> Abs1/1, Sign1/1, Product11/2, Product11/1
  Constant26/1 -> Product12/1
  Abs1/1 -> Product12/2
  Product12/1 -> Add7/1
  Product11/1 -> Add7/2
  Add7/1 -> Product13/2
  Product13/1 -> Out1/1
  Sign1/1 -> Product13/1

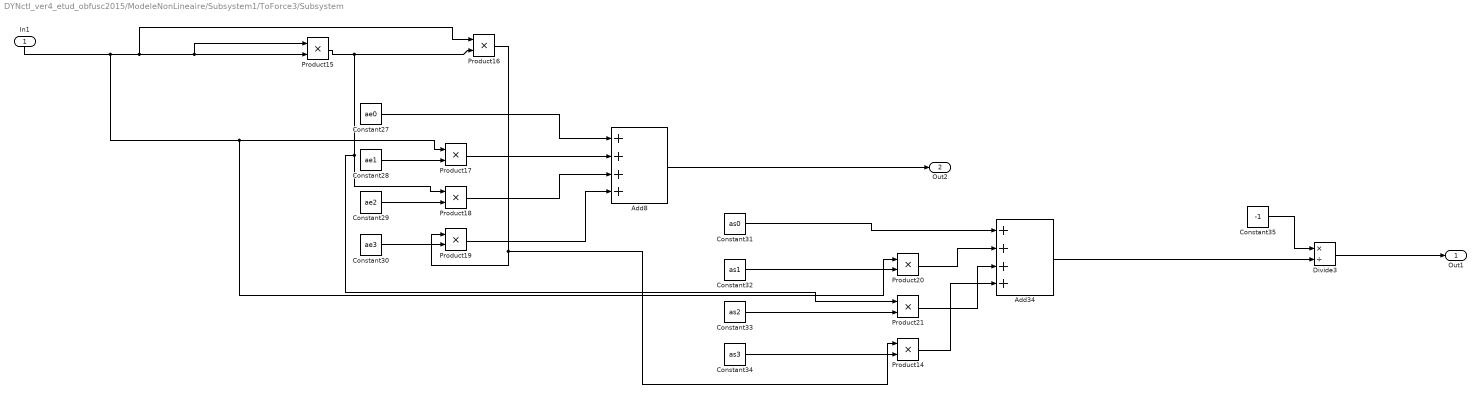
== system DYNctl_ver4_etud_obfusc2015/ModeleNonLineaire/Subsystem1/ToForce3/Subsystem ==
  In1 : Inport
  Add34 : Sum  Inputs=++++
  Add8 : Sum  Inputs=++++
  Constant27 : Constant  Value=ae0
  Constant28 : Constant  Value=ae1
  Constant29 : Constant  Value=ae2
  Constant30 : Constant  Value=ae3
  Constant31 : Constant  Value=as0
  Constant32 : Constant  Value=as1
  Constant33 : Constant  Value=as2
  Constant34 : Constant  Value=as3
  Constant35 : Constant  Value=-1
  Divide3 : Product  Inputs=*/
  Product{14..21} (8 alike) : Product
  Out1 : Outport
  Out2 : Outport  Port=2
  wires:
  In1/1 -> Product20/1, Product17/1, Product16/1, Product15/1, Product15/2
  Constant28/1 -> Product17/2
  Constant30/1 -> Product19/2
  Constant29/1 -> Product18/2
  Product15/1 -> Product21/1, Product18/1, Product16/2
  Product16/1 -> Product19/1, Product14/1
  Constant27/1 -> Add8/1
  Product17/1 -> Add8/2
  Product18/1 -> Add8/3
  Product19/1 -> Add8/4
  Add8/1 -> Out2/1
  Constant34/1 -> Product14/2
  Constant32/1 -> Product20/2
  Constant33/1 -> Product21/2
  Product20/1 -> Add34/2
  Product21/1 -> Add34/3
  Product14/1 -> Add34/4
  Constant31/1 -> Add34/1
  Add34/1 -> Divide3/2
  Constant35/1 -> Divide3/1
  Divide3/1 -> Out1/1

== system DYNctl_ver4_etud_obfusc2015/ModeleNonLineaire/Subsystem1/ToForce3/Subsystem1 ==
  In1 : Inport
  Abs1 : Abs
  Add7 : Sum
  Constant26 : Constant  Value=be1
  Product11 : Product
  Product12 : Product
  Product13 : Product
  Sign1 : Signum
  Out1 : Outport
  wires:
  In1/1 -> Abs1/1, Sign1/1, Product11/2, Product11/1
  Constant26/1 -> Product12/1
  Abs1/1 -> Product12/2
  Product12/1 -> Add7/1
  Product11/1 -> Add7/2
  Add7/1 -> Product13/2
  Product13/1 -> Out1/1
  Sign1/1 -> Product13/1
